simulink model "EGRVlv_VDPosGov"  (R2018a)
settings: configuration reference "cs_ert" (kept outside this file)
model workspace (MAT data in the model file):
  EGRVlv_VDPosGov_DT = 10
values from neighbouring files (symbols this model uses):
  EGRVlv_DKdNgv_C = -5.0    [EGRVlv_VDPosGov.sldd]
  EGRVlv_DKdPsv_C = 5.0    [EGRVlv_VDPosGov.sldd]
  EGRVlv_facCrntEffFlt_C = 50.0    [EGRVlv_VDPosGov.sldd]
  EGRVlv_iEff_CUR : value not decoded    [EGRVlv_VDPosGov.sldd]
  EGRVlv_iEff_CURX : value not decoded    [EGRVlv_VDPosGov.sldd]
  EGRVlv_iEffOvrLd_C = 200.0    [EGRVlv_VDPosGov.sldd]
  EGRVlv_rDesEGR_CUR : value not decoded    [EGRVlv_VDPosGov.sldd]
  EGRVlv_rDesEGR_CURX : value not decoded    [EGRVlv_VDPosGov.sldd]
  EGRVlv_rEGRDflVal_C = 0.0    [EGRVlv_VDPosGov.sldd]
  EGRVlv_rEGRSwtOff_C = 20.0    [EGRVlv_VDPosGov.sldd]
  EGRVlv_rGovDvtThres_C = 30.0    [EGRVlv_VDPosGov.sldd]
  EGRVlv_rGovMax_C = 30.0    [EGRVlv_VDPosGov.sldd]
  EGRVlv_rGovMax_CUR : value not decoded    [EGRVlv_VDPosGov.sldd]
  EGRVlv_rGovMax_CURX : value not decoded    [EGRVlv_VDPosGov.sldd]
  EGRVlv_rGovMin_C = 10.0    [EGRVlv_VDPosGov.sldd]
  EGRVlv_rGovMin_CUR : value not decoded    [EGRVlv_VDPosGov.sldd]
  EGRVlv_rGovMin_CURX : value not decoded    [EGRVlv_VDPosGov.sldd]
  EGRVlv_rIniStp_C = 5.0    [EGRVlv_VDPosGov.sldd]
  EGRVlv_rOutIMax_C = 30.0    [EGRVlv_VDPosGov.sldd]
  EGRVlv_rPIDWinNgv_C = -10.0    [EGRVlv_VDPosGov.sldd]
  EGRVlv_rPIDWinPsv_C = 10.0    [EGRVlv_VDPosGov.sldd]
  EGRVlv_rSwtOffRmp_C = 2.0    [EGRVlv_VDPosGov.sldd]
  EGRVlv_SlwClsDKd_C = 3.0    [EGRVlv_VDPosGov.sldd]
  EGRVlv_SlwClsIKi_C = 0.2    [EGRVlv_VDPosGov.sldd]
  EGRVlv_SlwClsPKp_C = 3.0    [EGRVlv_VDPosGov.sldd]
  EGRVlv_SmlSigNgvDKd_C = -5.0    [EGRVlv_VDPosGov.sldd]
  EGRVlv_SmlSigNgvIKi_C = -1.0    [EGRVlv_VDPosGov.sldd]
  EGRVlv_SmlSigNgvPKp_C = -5.0    [EGRVlv_VDPosGov.sldd]
  EGRVlv_SmlSigPsvDKd_C = 5.0    [EGRVlv_VDPosGov.sldd]
  EGRVlv_SmlSigPsvIKi_C = 1.0    [EGRVlv_VDPosGov.sldd]
  EGRVlv_SmlSigPsvPKp_C = 5.0    [EGRVlv_VDPosGov.sldd]
  EGRVlv_swtDesValNrmInv_C = 1.0    [EGRVlv_VDPosGov.sldd]
  EGRVlv_swtGovByp_C = 0.0    [EGRVlv_VDPosGov.sldd]
  EGRVlv_tiLimDlyOvrLd_C = 1.0    [EGRVlv_VDPosGov.sldd]
  EGRVlv_tiOutIMax_C = 1.0    [EGRVlv_VDPosGov.sldd]
undefined symbols (not defined in the file or in its folder): CEngDsT_tTransf_CURX
libraries: simulink x10, sllib x5
settings Model: DataDictionary=EGRVlv_VDPosGov.sldd  Creator=zhoutinglin  LastModifiedBy=zhoutinglin

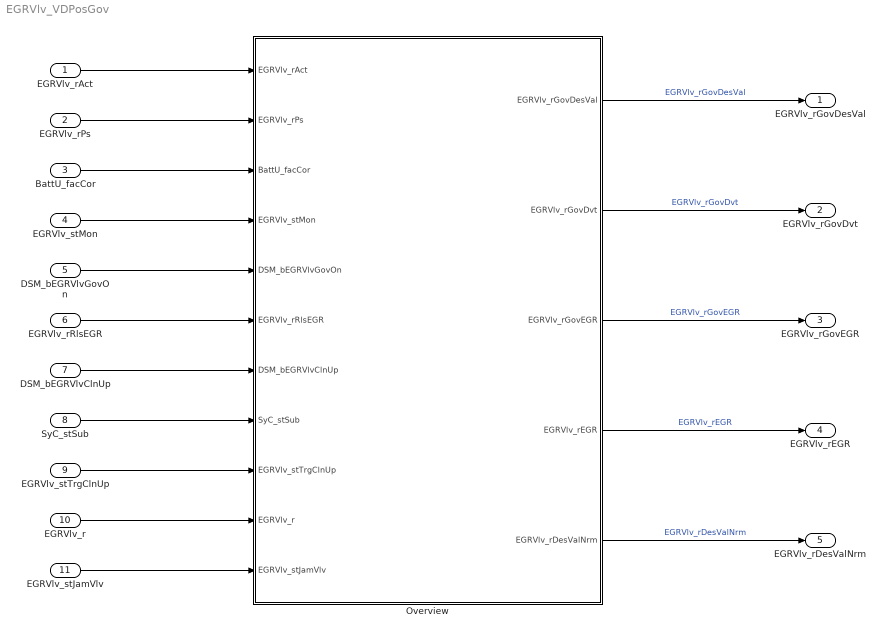
== system EGRVlv_VDPosGov ==
  EGRVlv_rAct : Inport  Description=Commanded value from application SW  OutMin=-100  OutMax=100  OutDataTypeStr=DutyCycle  Unit=%  PortDimensions=[1 1]
  EGRVlv_rPs : Inport  Description=Actuatorposition  Port=2  OutMin=-100  OutMax=100  OutDataTypeStr=DutyCycle  Unit=%  PortDimensions=[1 1]
  BattU_facCor : Inport  Description=Additional control value to release a jammed valve  Port=3  OutMin=-32  OutMax=31.9  OutDataTypeStr=Fac_100  PortDimensions=[1 1]
  EGRVlv_stMon : Inport  Description=Duty cycle to power stage  Port=4  OutMin=0  OutMax=65535  OutDataTypeStr=State2  PortDimensions=[1 1]
  DSM_bEGRVlvGovOn : Inport  Description=Battery correction factor  Port=5  OutMin=0  OutMax=1  OutDataTypeStr=boolean  PortDimensions=[1 1]
  EGRVlv_rRlsEGR : Inport  Description=State of system monitoring  Port=6  OutMin=-100  OutMax=100  OutDataTypeStr=DutyCycle  PortDimensions=[1 1]
  DSM_bEGRVlvClnUp : Inport  Description=Status of FId_EGRVlvGovOn  Port=7  OutMin=0  OutMax=1  OutDataTypeStr=boolean  PortDimensions=[1 1]
  SyC_stSub : Inport  Description=Status of offset learning  Port=8  OutDataTypeStr=Enum: ECUPowerState  PortDimensions=[1 1]
  EGRVlv_stTrgClnUp : Inport  Description=Valve position (offset corrected without error handling)  Port=9  OutMin=0  OutMax=1  OutDataTypeStr=boolean  PortDimensions=[1 1]
  EGRVlv_r : Inport  Description=Status of FId_EGRVlvClnUp  Port=10  OutMin=-100  OutMax=100  OutDataTypeStr=DutyCycle  PortDimensions=[1 1]
  EGRVlv_stJamVlv : Inport  Description=Current system/ECU sub-state  Port=11  OutMin=0  OutMax=1  OutDataTypeStr=boolean  PortDimensions=[1 1]
  Overview : Subsystem
  EGRVlv_rGovDesVal : Outport
  EGRVlv_rGovDvt : Outport  Port=2
  EGRVlv_rGovEGR : Outport  Port=3
  EGRVlv_rEGR : Outport  Port=4
  EGRVlv_rDesValNrm : Outport  Port=5
  wires:
  EGRVlv_rAct/1 -> Overview/1(EGRVlv_rAct)
  EGRVlv_rPs/1 -> Overview/2(EGRVlv_rPs)
  BattU_facCor/1 -> Overview/3(BattU_facCor)
  EGRVlv_stMon/1 -> Overview/4(EGRVlv_stMon)
  DSM_bEGRVlvGovOn/1 -> Overview/5(DSM_bEGRVlvGovOn)
  EGRVlv_rRlsEGR/1 -> Overview/6(EGRVlv_rRlsEGR)
  DSM_bEGRVlvClnUp/1 -> Overview/7(DSM_bEGRVlvClnUp)
  SyC_stSub/1 -> Overview/8(SyC_stSub)
  EGRVlv_stTrgClnUp/1 -> Overview/9(EGRVlv_stTrgClnUp)
  EGRVlv_r/1 -> Overview/10(EGRVlv_r)
  EGRVlv_stJamVlv/1 -> Overview/11(EGRVlv_stJamVlv)
  Overview/1(EGRVlv_rGovDesVal) -> EGRVlv_rGovDesVal/1  "EGRVlv_rGovDesVal"
  Overview/2(EGRVlv_rGovDvt) -> EGRVlv_rGovDvt/1  "EGRVlv_rGovDvt"
  Overview/3(EGRVlv_rGovEGR) -> EGRVlv_rGovEGR/1  "EGRVlv_rGovEGR"
  Overview/4(EGRVlv_rEGR) -> EGRVlv_rEGR/1  "EGRVlv_rEGR"
  Overview/5(EGRVlv_rDesValNrm) -> EGRVlv_rDesValNrm/1  "EGRVlv_rDesValNrm"

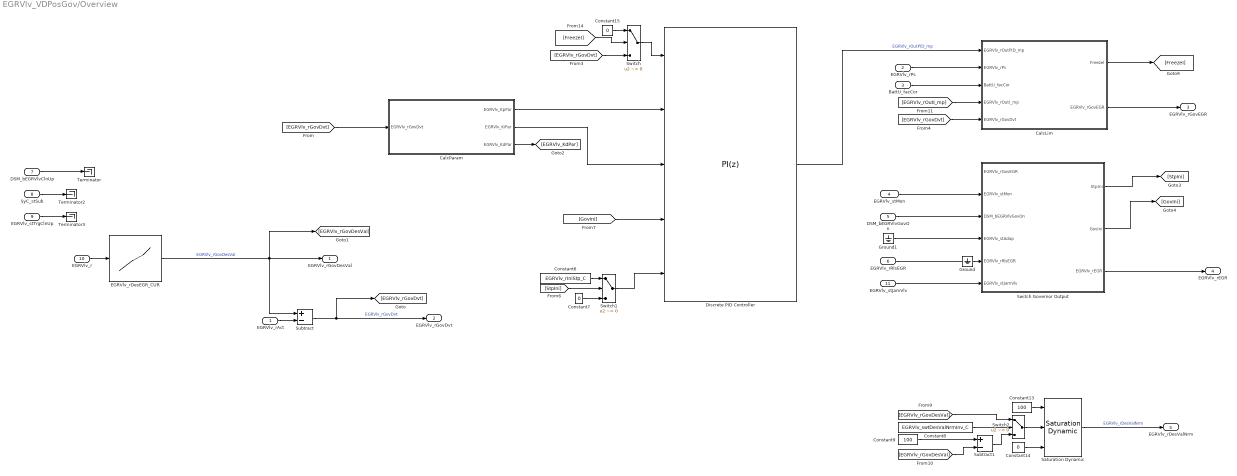
== system EGRVlv_VDPosGov/Overview ==
  EGRVlv_rAct : Inport  Tag=%
  EGRVlv_rPs : Inport  Tag=%  Port=2
  BattU_facCor : Inport  Tag=%  Port=3
  EGRVlv_stMon : Inport  Tag=%  Port=4
  DSM_bEGRVlvGovOn : Inport  Tag=%  Port=5
  EGRVlv_rRlsEGR : Inport  Tag=%  Port=6
  DSM_bEGRVlvClnUp : Inport  Tag=%  Port=7
  SyC_stSub : Inport  Tag=%  Port=8
  EGRVlv_stTrgClnUp : Inport  Tag=%  Port=9
  EGRVlv_r : Inport  Tag=%  Port=10
  EGRVlv_stJamVlv : Inport  Port=11
  CalcLim : Subsystem
  CalcParam : Subsystem
  Constant13 : Constant  Value=100  OutDataTypeStr=Inherit: Inherit via back propagation
  Constant14 : Constant  Value=0  OutDataTypeStr=Inherit: Inherit via back propagation
  Constant15 : Constant  Value=0  OutDataTypeStr=Inherit: Inherit via back propagation
  Constant6 : Constant  Value=EGRVlv_rIniStp_C
  Constant7 : Constant  Value=0  OutDataTypeStr=Inherit: Inherit via back propagation
  Constant8 : Constant  Value=EGRVlv_swtDesValNrmInv_C
  Constant9 : Constant  Value=100  OutDataTypeStr=Inherit: Inherit via back propagation
  Discrete PID Controller : simulink/Continuous/PID Controller  Controller=PI  TimeDomain=Discrete-time  SampleTime=-1  IntegratorMethod=Forward Euler  FilterMethod=Forward Euler  Form=Parallel  UseFilter=on  ControllerParametersSource=external  P=1  I=1  D=0  N=100  InitialConditionSource=external  InitialConditionForIntegrator=0  InitialConditionForFilter=0  ExternalReset=level  ZeroCross=off  LimitOutput=off  UpperSaturationLimit=inf  LowerSaturationLimit=-inf  LinearizeAsGain=off  AntiWindupMode=none  Kb=1  TrackingMode=off  Kt=1  SaturateOnIntegerOverflow=on  PParamMin=[]  PParamMax=[]  IParamMin=[]  IParamMax=[]  DParamMin=[]  DParamMax=[]  NParamMin=[]  NParamMax=[]  KbParamMin=[]  KbParamMax=[]  KtParamMin=[]  KtParamMax=[]  POutMin=[]  POutMax=[]  IOutMin=[]  IOutMax=[]  DOutMin=[]  DOutMax=[]  NOutMin=[]  NOutMax=[]  KbOutMin=[]  KbOutMax=[]  KtOutMin=[]  KtOutMax=[]  IntegratorOutMin=[]  IntegratorOutMax=[]  FilterOutMin=[]  FilterOutMax=[]  SumOutMin=[]  SumOutMax=[]  SumOutDataTypeStr=Inherit: Inherit via back propagation  SumI1OutMin=[]  SumI1OutMax=[]  SumI2OutMin=[]  SumI2OutMax=[]  SumI3OutMin=[]  SumI3OutMax=[]  SumDOutMin=[]  SumDOutMax=[]  SaturationOutMin=[]  SaturationOutMax=[]  IntegratorContinuousStateAttributes=''  IntegratorStateMustResolveToSignalObject=off  IntegratorRTWStateStorageClass=Auto  FilterContinuousStateAttributes=''  FilterStateMustResolveToSignalObject=off  FilterRTWStateStorageClass=Auto  DifferentiatorICPrevScaledInput=0  DifferentiatorOutMin=[]  DifferentiatorOutMax=[]  FilterDiffOutCoefMin=[]  FilterDiffOutCoefMax=[]  SumDenOutMin=[]  SumDenOutMax=[]  SumNumOutMin=[]  SumNumOutMax=[]  ReciprocalOutMin=[]  ReciprocalOutMax=[]  DivideOutMin=[]  DivideOutMax=[]  TunerSelectOption=Transfer Function Based (PID Tuner App)
  EGRVlv_rDesEGR_CUR : Lookup_n-D  DialogController=Simulink.DDGSource  NumberOfTableDimensions=1  BreakpointsForDimension1=EGRVlv_rDesEGR_CURX  BreakpointsForDimension2=CEngDsT_tTransf_CURX  IndexSearchMethod=Linear search  BeginIndexSearchUsingPreviousIndexResult=on  Table=EGRVlv_rDesEGR_CUR  TableDataTypeStr=Inherit: Inherit from 'Table data'  ExtrapMethod=Clip  UseLastTableValue=on  InternalRulePriority=Speed  OutDataTypeStr=Inherit: Inherit from 'Table data'  SaturateOnIntegerOverflow=on
  Ground : Ground
  Ground1 : Ground
  Saturation Dynamic : simulink/Discontinuities/Saturation Dynamic  OutMin=[]  OutMax=[]  OutDataTypeStr=Inherit: Same as second input  OutDataType=fixdt(1, 16)  OutScaling=2^-10  DoSatur=off
  Subtract : Sum  Inputs=+-  SaturateOnIntegerOverflow=on
  Subtract1 : Sum  Inputs=+-  SaturateOnIntegerOverflow=on  InputSameDT=on
  Switch : Switch  Criteria=u2 ~= 0
  Switch Governor Output : Subsystem
  Switch1 : Switch  Criteria=u2 ~= 0
  Switch2 : Switch  Criteria=u2 ~= 0  InputSameDT=on
  Terminator : Terminator
  Terminator2 : Terminator
  Terminator3 : Terminator
  EGRVlv_rGovDesVal : Outport  Tag=%
  EGRVlv_rGovDvt : Outport  Tag=%  Port=2
  EGRVlv_rGovEGR : Outport  Tag=%  Port=3
  EGRVlv_rEGR : Outport  Tag=%  Port=4
  EGRVlv_rDesValNrm : Outport  Tag=%  Port=5
  wires:
  [EGRVlv_rGovDvt] -> CalcLim/5(EGRVlv_rGovDvt)
  CalcParam/1(EGRVlv_KpPar) -> Discrete PID Controller/2
  Saturation Dynamic/1 -> EGRVlv_rDesValNrm/1  "EGRVlv_rDesValNrm"
  CalcLim/1(Freezel) -> [FreezeI]
  Switch1/1 -> Discrete PID Controller/5
  Switch/1 -> Discrete PID Controller/1
  Constant14/1 -> Saturation Dynamic/3
  [GovIni] -> Discrete PID Controller/4
  Subtract1/1 -> Switch2/3
  Switch2/1 -> Saturation Dynamic/2
  [FreezeI] -> Switch/2
  Switch Governor Output/2(GovIni) -> [GovIni]
  [EGRVlv_rGovDvt] -> CalcParam/1(EGRVlv_rGovDvt)
  [EGRVlv_rOutI_mp] -> CalcLim/4(EGRVlv_rOutI_mp)
  Switch Governor Output/1(StpIni) -> [StpIni]
  DSM_bEGRVlvClnUp/1 -> Terminator/1
  Constant9/1 -> Subtract1/1
  SyC_stSub/1 -> Terminator2/1
  EGRVlv_stTrgClnUp/1 -> Terminator3/1
  Constant15/1 -> Switch/1
  [StpIni] -> Switch1/2
  Constant6/1 -> Switch1/1
  Constant7/1 -> Switch1/3
  Constant13/1 -> Saturation Dynamic/1
  Discrete PID Controller/1 -> CalcLim/1(EGRVlv_rOutPID_mp)  "EGRVlv_rOutPID_mp"
  CalcParam/3(EGRVlv_KdPar) -> [EGRVlv_KdPar]
  EGRVlv_rDesEGR_CUR/1 -> [EGRVlv_rGovDesVal], EGRVlv_rGovDesVal/1, Subtract/1  "EGRVlv_rGovDesVal"
  [EGRVlv_rGovDesVal] -> Subtract1/2
  CalcParam/2(EGRVlv_KiPar) -> Discrete PID Controller/3
  [EGRVlv_rGovDesVal] -> Switch2/1
  [EGRVlv_rGovDvt] -> Switch/3
  BattU_facCor/1 -> CalcLim/3(BattU_facCor)
  CalcLim/2(EGRVlv_rGovEGR) -> EGRVlv_rGovEGR/1
  EGRVlv_rPs/1 -> CalcLim/2(EGRVlv_rPs)
  EGRVlv_rAct/1 -> Subtract/2
  Subtract/1 -> EGRVlv_rGovDvt/1, [EGRVlv_rGovDvt]  "EGRVlv_rGovDvt"
  Constant8/1 -> Switch2/2
  EGRVlv_r/1 -> EGRVlv_rDesEGR_CUR/1
  Ground/1 -> ?
  EGRVlv_stMon/1 -> Switch Governor Output/2(EGRVlv_stMon)
  DSM_bEGRVlvGovOn/1 -> Switch Governor Output/3(DSM_bEGRVlvGovOn)
  Ground1/1 -> Switch Governor Output/4(EGRVlv_stAdap)
  EGRVlv_rRlsEGR/1 -> Switch Governor Output/5(EGRVlv_rRlsEGR)
  EGRVlv_stJamVlv/1 -> Switch Governor Output/6(EGRVlv_stJamVlv)
  Switch Governor Output/3(EGRVlv_rEGR) -> EGRVlv_rEGR/1

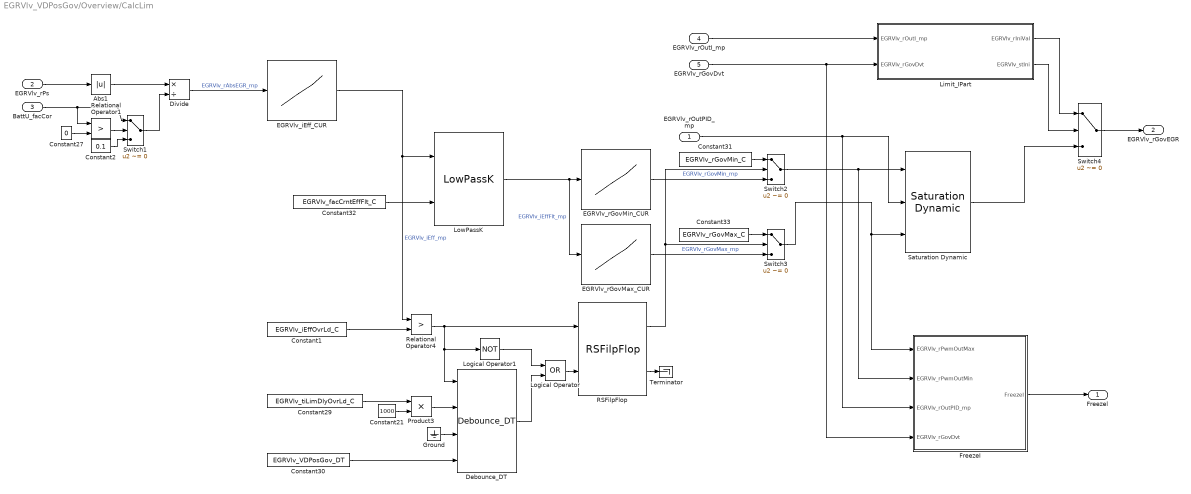
== system EGRVlv_VDPosGov/Overview/CalcLim ==
  EGRVlv_rOutPID_mp : Inport  Tag=%
  EGRVlv_rPs : Inport  Tag=%  Port=2
  BattU_facCor : Inport  Tag=%  Port=3
  EGRVlv_rOutI_mp : Inport  Tag=%  Port=4
  EGRVlv_rGovDvt : Inport  Tag=%  Port=5
  Abs1 : Abs
  Constant1 : Constant  Value=EGRVlv_iEffOvrLd_C
  Constant2 : Constant  Value=0.1  OutDataTypeStr=Inherit: Inherit via back propagation
  Constant21 : Constant  Value=1000  OutDataTypeStr=uint16
  Constant27 : Constant  Value=0  OutDataTypeStr=Inherit: Inherit via back propagation
  Constant29 : Constant  Value=EGRVlv_tiLimDlyOvrLd_C
  Constant30 : Constant  Value=EGRVlv_VDPosGov_DT  OutDataTypeStr=Inherit: Inherit via back propagation
  Constant31 : Constant  Value=EGRVlv_rGovMin_C
  Constant32 : Constant  Value=EGRVlv_facCrntEffFlt_C
  Constant33 : Constant  Value=EGRVlv_rGovMax_C
  Debounce_DT : sllib/Debounce_DT
      settings: SourceProductName=sllib
  Divide : Product  Inputs=*/  OutDataTypeStr=Inherit: Inherit via back propagation  SaturateOnIntegerOverflow=on
  EGRVlv_iEff_CUR : Lookup_n-D  DialogController=Simulink.DDGSource  NumberOfTableDimensions=1  BreakpointsForDimension1=EGRVlv_iEff_CURX  BreakpointsForDimension2=CEngDsT_tTransf_CURX  IndexSearchMethod=Linear search  BeginIndexSearchUsingPreviousIndexResult=on  Table=EGRVlv_iEff_CUR  TableDataTypeStr=Inherit: Inherit from 'Table data'  ExtrapMethod=Clip  UseLastTableValue=on  InternalRulePriority=Speed  OutDataTypeStr=Inherit: Inherit from 'Table data'  SaturateOnIntegerOverflow=on
  EGRVlv_rGovMax_CUR : Lookup_n-D  DialogController=Simulink.DDGSource  NumberOfTableDimensions=1  BreakpointsForDimension1=EGRVlv_rGovMax_CURX  BreakpointsForDimension2=CEngDsT_tTransf_CURX  IndexSearchMethod=Linear search  BeginIndexSearchUsingPreviousIndexResult=on  Table=EGRVlv_rGovMax_CUR  TableDataTypeStr=Inherit: Inherit from 'Table data'  ExtrapMethod=Clip  UseLastTableValue=on  InternalRulePriority=Speed  OutDataTypeStr=Inherit: Inherit from 'Table data'  SaturateOnIntegerOverflow=on
  EGRVlv_rGovMin_CUR : Lookup_n-D  DialogController=Simulink.DDGSource  NumberOfTableDimensions=1  BreakpointsForDimension1=EGRVlv_rGovMin_CURX  BreakpointsForDimension2=CEngDsT_tTransf_CURX  IndexSearchMethod=Linear search  BeginIndexSearchUsingPreviousIndexResult=on  Table=EGRVlv_rGovMin_CUR  TableDataTypeStr=Inherit: Inherit from 'Table data'  ExtrapMethod=Clip  UseLastTableValue=on  InternalRulePriority=Speed  OutDataTypeStr=Inherit: Inherit from 'Table data'  SaturateOnIntegerOverflow=on
  FreezeI : Subsystem
  Ground : Ground
  Limit_IPart : Subsystem
  Logical Operator : Logic  Operator=OR  AllPortsSameDT=off  OutDataTypeStr=boolean
  Logical Operator1 : Logic  Operator=NOT  AllPortsSameDT=off  OutDataTypeStr=boolean
  LowPassK : sllib/LowPassK
      settings: SourceProductName=sllib
  Product3 : Product  OutDataTypeStr=uint32  SaturateOnIntegerOverflow=on
  RSFilpFlop : sllib/RSFilpFlop
      settings: SourceProductName=sllib
  Relational Operator1 : RelationalOperator  Operator=>  OutDataTypeStr=boolean  RndMeth=Simplest  InputSameDT=on
  Relational Operator4 : RelationalOperator  Operator=>  OutDataTypeStr=boolean  RndMeth=Simplest
  Saturation Dynamic : simulink/Discontinuities/Saturation Dynamic  OutMin=[]  OutMax=[]  OutDataTypeStr=Inherit: Same as second input  OutDataType=fixdt(1, 16)  OutScaling=2^-10  DoSatur=off
  Switch{1..4} (4 alike) : Switch  Criteria=u2 ~= 0
  Terminator : Terminator
  Freezel : Outport
  EGRVlv_rGovEGR : Outport  Tag=%  Port=2
  wires:
  Abs1/1 -> Divide/1
  Constant33/1 -> Switch3/1
  RSFilpFlop/1 -> Switch3/2, Switch2/2
  EGRVlv_rGovMax_CUR/1 -> Switch3/3  "EGRVlv_rGovMax_mp"
  Switch2/1 -> Saturation Dynamic/1, FreezeI/2(EGRVlv_rPwmOutMin)
  Switch3/1 -> Saturation Dynamic/3, FreezeI/1(EGRVlv_rPwmOutMax)
  Debounce_DT/1 -> Logical Operator/2
  Logical Operator/1 -> RSFilpFlop/2
  Logical Operator1/1 -> Logical Operator/1
  Constant31/1 -> Switch2/1
  EGRVlv_iEff_CUR/1 -> Relational Operator4/1, LowPassK/1  "EGRVlv_iEff_mp"
  EGRVlv_rGovMin_CUR/1 -> Switch2/3  "EGRVlv_rGovMin_mp"
  Constant1/1 -> Relational Operator4/2
  Relational Operator4/1 -> RSFilpFlop/1, Debounce_DT/1, Logical Operator1/1
  EGRVlv_rPs/1 -> Abs1/1
  Divide/1 -> EGRVlv_iEff_CUR/1  "EGRVlv_rAbsEGR_mp"
  LowPassK/1 -> EGRVlv_rGovMax_CUR/1, EGRVlv_rGovMin_CUR/1  "EGRVlv_iEffFlt_mp"
  Constant29/1 -> Product3/1
  Constant30/1 -> Debounce_DT/4
  BattU_facCor/1 -> Relational Operator1/1, Switch1/1
  Constant32/1 -> LowPassK/2
  Relational Operator1/1 -> Switch1/2
  Constant27/1 -> Relational Operator1/2
  Constant2/1 -> Switch1/3
  Switch1/1 -> Divide/2
  Product3/1 -> Debounce_DT/2
  Limit_IPart/1(EGRVlv_rIniVal) -> Switch4/1
  Limit_IPart/2(EGRVlv_stIni) -> Switch4/2
  Switch4/1 -> EGRVlv_rGovEGR/1
  Saturation Dynamic/1 -> Switch4/3
  Constant21/1 -> Product3/2
  EGRVlv_rOutPID_mp/1 -> Saturation Dynamic/2, FreezeI/3(EGRVlv_rOutPID_mp)
  RSFilpFlop/2 -> Terminator/1
  EGRVlv_rOutI_mp/1 -> Limit_IPart/1(EGRVlv_rOutI_mp)
  EGRVlv_rGovDvt/1 -> Limit_IPart/2(EGRVlv_rGovDvt), FreezeI/4(EGRVlv_rGovDvt)
  FreezeI/1(FreezeI) -> Freezel/1
  Ground/1 -> Debounce_DT/3

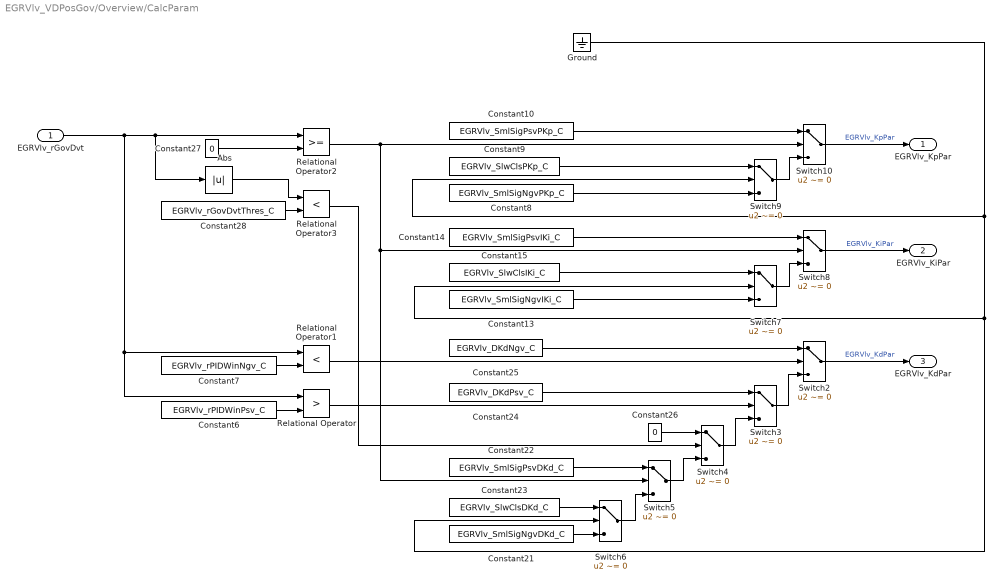
== system EGRVlv_VDPosGov/Overview/CalcParam ==
  EGRVlv_rGovDvt : Inport  Tag=%
  Abs : Abs
  Constant10 : Constant  Value=EGRVlv_SmlSigPsvPKp_C
  Constant13 : Constant  Value=EGRVlv_SmlSigNgvIKi_C
  Constant14 : Constant  Value=EGRVlv_SmlSigPsvIKi_C
  Constant15 : Constant  Value=EGRVlv_SlwClsIKi_C
  Constant21 : Constant  Value=EGRVlv_SmlSigNgvDKd_C
  Constant22 : Constant  Value=EGRVlv_SmlSigPsvDKd_C
  Constant23 : Constant  Value=EGRVlv_SlwClsDKd_C
  Constant24 : Constant  Value=EGRVlv_DKdPsv_C
  Constant25 : Constant  Value=EGRVlv_DKdNgv_C
  Constant26 : Constant  Value=0  OutDataTypeStr=Inherit: Inherit via back propagation
  Constant27 : Constant  Value=0  OutDataTypeStr=Inherit: Inherit via back propagation
  Constant28 : Constant  Value=EGRVlv_rGovDvtThres_C
  Constant6 : Constant  Value=EGRVlv_rPIDWinPsv_C
  Constant7 : Constant  Value=EGRVlv_rPIDWinNgv_C
  Constant8 : Constant  Value=EGRVlv_SmlSigNgvPKp_C
  Constant9 : Constant  Value=EGRVlv_SlwClsPKp_C
  Ground : Ground
  Relational Operator : RelationalOperator  Operator=>  OutDataTypeStr=boolean  RndMeth=Simplest
  Relational Operator1 : RelationalOperator  Operator=<  OutDataTypeStr=boolean  RndMeth=Simplest
  Relational Operator2 : RelationalOperator  OutDataTypeStr=boolean  RndMeth=Simplest  InputSameDT=on
  Relational Operator3 : RelationalOperator  Operator=<  OutDataTypeStr=boolean  RndMeth=Simplest
  Switch{2..10} (9 alike) : Switch  Criteria=u2 ~= 0
  EGRVlv_KpPar : Outport  Tag=%
  EGRVlv_KiPar : Outport  Tag=%  Port=2
  EGRVlv_KdPar : Outport  Tag=%  Port=3
  wires:
  Constant6/1 -> Relational Operator/2
  EGRVlv_rGovDvt/1 -> Relational Operator2/1, Abs/1, Relational Operator1/1, Relational Operator/1
  Constant7/1 -> Relational Operator1/2
  Abs/1 -> Relational Operator3/1
  Constant27/1 -> Relational Operator2/2
  Constant28/1 -> Relational Operator3/2
  Relational Operator1/1 -> Switch2/2
  Constant25/1 -> Switch2/1
  Switch3/1 -> Switch2/3
  Relational Operator/1 -> Switch3/2
  Constant24/1 -> Switch3/1
  Switch4/1 -> Switch3/3
  Relational Operator3/1 -> Switch4/2
  Constant26/1 -> Switch4/1
  Switch5/1 -> Switch4/3
  Relational Operator2/1 -> Switch10/2, Switch8/2, Switch5/2
  Constant22/1 -> Switch5/1
  Switch6/1 -> Switch5/3
  Constant23/1 -> Switch6/1
  Constant21/1 -> Switch6/3
  Switch7/1 -> Switch8/3
  Constant14/1 -> Switch8/1
  Constant15/1 -> Switch7/1
  Constant13/1 -> Switch7/3
  Ground/1 -> Switch6/2, Switch7/2, Switch9/2
  Switch9/1 -> Switch10/3
  Constant10/1 -> Switch10/1
  Constant9/1 -> Switch9/1
  Constant8/1 -> Switch9/3
  Switch10/1 -> EGRVlv_KpPar/1  "EGRVlv_KpPar"
  Switch8/1 -> EGRVlv_KiPar/1  "EGRVlv_KiPar"
  Switch2/1 -> EGRVlv_KdPar/1  "EGRVlv_KdPar"

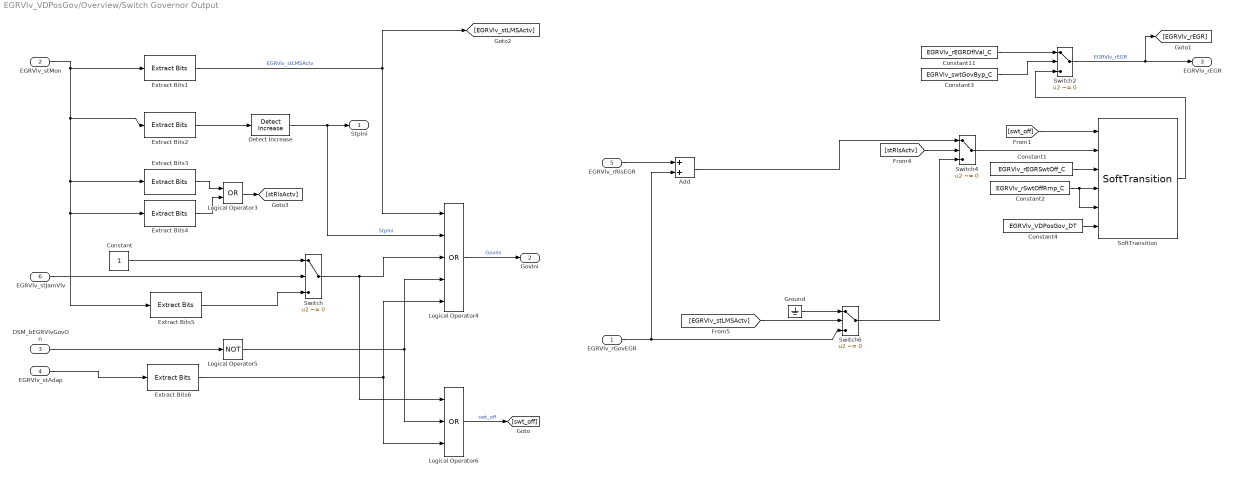
== system EGRVlv_VDPosGov/Overview/Switch Governor Output ==
  EGRVlv_rGovEGR : Inport  Tag=%
  EGRVlv_stMon : Inport  Tag=%  Port=2
  DSM_bEGRVlvGovOn : Inport  Tag=%  Port=3
  EGRVlv_stAdap : Inport  Tag=%  Port=4
  EGRVlv_rRlsEGR : Inport  Tag=%  Port=5
  EGRVlv_stJamVlv : Inport  Port=6
  Add : Sum  SaturateOnIntegerOverflow=on
  Constant : Constant  OutDataTypeStr=boolean
  Constant1 : Constant  Value=EGRVlv_rEGRSwtOff_C
  Constant11 : Constant  Value=EGRVlv_rEGRDflVal_C
  Constant2 : Constant  Value=EGRVlv_rSwtOffRmp_C
  Constant3 : Constant  Value=EGRVlv_swtGovByp_C
  Constant4 : Constant  Value=EGRVlv_VDPosGov_DT  OutDataTypeStr=Inherit: Inherit via back propagation
  Detect Increase : simulink/Logic and Bit Operations/Detect Increase  vinit=0.0  OutDataTypeStr=boolean
  Extract Bits1 : simulink/Logic and Bit Operations/Extract Bits  bitsToExtract=Range of bits  numBits=8  bitIdxRange=[0 0]  outScalingMode=Treat bit field as an integer
      settings: SourceProductName=Simulink
  Extract Bits2 : simulink/Logic and Bit Operations/Extract Bits  bitsToExtract=Range of bits  numBits=8  bitIdxRange=[4 4]  outScalingMode=Treat bit field as an integer
      settings: SourceProductName=Simulink
  Extract Bits3 : simulink/Logic and Bit Operations/Extract Bits  bitsToExtract=Range of bits  numBits=8  bitIdxRange=[6 6]  outScalingMode=Treat bit field as an integer
      settings: SourceProductName=Simulink
  Extract Bits4 : simulink/Logic and Bit Operations/Extract Bits  bitsToExtract=Range of bits  numBits=8  bitIdxRange=[8 8]  outScalingMode=Treat bit field as an integer
      settings: SourceProductName=Simulink
  Extract Bits5 : simulink/Logic and Bit Operations/Extract Bits  bitsToExtract=Range of bits  numBits=8  bitIdxRange=[10 10]  outScalingMode=Treat bit field as an integer
      settings: SourceProductName=Simulink
  Extract Bits6 : simulink/Logic and Bit Operations/Extract Bits  bitsToExtract=Range of bits  numBits=8  bitIdxRange=[0 0]  outScalingMode=Treat bit field as an integer
      settings: SourceProductName=Simulink
  Ground : Ground
  Logical Operator3 : Logic  Operator=OR  AllPortsSameDT=off  OutDataTypeStr=boolean
  Logical Operator4 : Logic  Operator=OR  Inputs=5  AllPortsSameDT=off  OutDataTypeStr=boolean
  Logical Operator5 : Logic  Operator=NOT  AllPortsSameDT=off  OutDataTypeStr=boolean
  Logical Operator6 : Logic  Operator=OR  Inputs=3  AllPortsSameDT=off  OutDataTypeStr=boolean
  SoftTransition : sllib/SoftTransition
      settings: SourceProductName=sllib
  Switch{,2,4,6} (4 alike) : Switch  Criteria=u2 ~= 0
  StpIni : Outport  Tag=%
  GovIni : Outport  Tag=%  Port=2
  EGRVlv_rEGR : Outport  Tag=%  Port=3
  wires:
  Logical Operator4/1 -> GovIni/1  "GovIni"
  Logical Operator5/1 -> Logical Operator4/4, Logical Operator6/2
  DSM_bEGRVlvGovOn/1 -> Logical Operator5/1
  Detect Increase/1 -> Logical Operator4/2, StpIni/1  "StpIni"
  Logical Operator6/1 -> [swt_off]  "swt_off"
  Extract Bits1/1 -> [EGRVlv_stLMSActv], Logical Operator4/1  "EGRVlv_stLMSActv"
  EGRVlv_rRlsEGR/1 -> Add/1
  EGRVlv_rGovEGR/1 -> Add/2, Switch6/3
  Switch2/1 -> EGRVlv_rEGR/1, [EGRVlv_rEGR]  "EGRVlv_rEGR"
  Constant2/1 -> SoftTransition/5, SoftTransition/4
  Ground/1 -> Switch6/1
  SoftTransition/1 -> Switch2/3
  Switch4/1 -> SoftTransition/2
  Switch6/1 -> Switch4/3
  Constant11/1 -> Switch2/1
  Constant3/1 -> Switch2/2
  [swt_off] -> SoftTransition/1
  Logical Operator3/1 -> [stRlsActv]
  [EGRVlv_stLMSActv] -> Switch6/2
  Extract Bits2/1 -> Detect Increase/1
  Extract Bits3/1 -> Logical Operator3/1
  Extract Bits4/1 -> Logical Operator3/2
  Extract Bits6/1 -> Logical Operator4/5, Logical Operator6/3
  EGRVlv_stMon/1 -> Extract Bits1/1, Extract Bits2/1, Extract Bits5/1, Extract Bits4/1, Extract Bits3/1
  Constant1/1 -> SoftTransition/3
  EGRVlv_stAdap/1 -> Extract Bits6/1
  [stRlsActv] -> Switch4/2
  Add/1 -> Switch4/1
  Constant/1 -> Switch/1
  EGRVlv_stJamVlv/1 -> Switch/2
  Extract Bits5/1 -> Switch/3
  Switch/1 -> Logical Operator6/1, Logical Operator4/3
  Constant4/1 -> SoftTransition/6

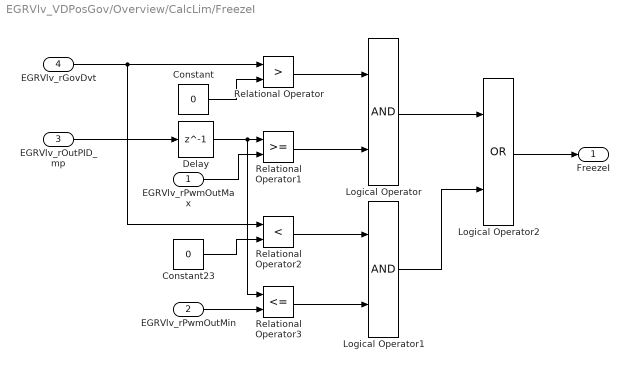
== system EGRVlv_VDPosGov/Overview/CalcLim/FreezeI ==
  EGRVlv_rPwmOutMax : Inport
  EGRVlv_rPwmOutMin : Inport  Port=2
  EGRVlv_rOutPID_mp : Inport  Port=3
  EGRVlv_rGovDvt : Inport  Port=4
  Constant : Constant  Value=0  OutDataTypeStr=Inherit: Inherit via back propagation
  Constant23 : Constant  Value=0  OutDataTypeStr=Inherit: Inherit via back propagation
  Delay : Delay  DelayLength=1  InitialCondition=0
  Logical Operator : Logic  AllPortsSameDT=off  OutDataTypeStr=boolean
  Logical Operator1 : Logic  AllPortsSameDT=off  OutDataTypeStr=boolean
  Logical Operator2 : Logic  Operator=OR  AllPortsSameDT=off  OutDataTypeStr=boolean
  Relational Operator : RelationalOperator  Operator=>  OutDataTypeStr=boolean  RndMeth=Simplest  InputSameDT=on
  Relational Operator1 : RelationalOperator  OutDataTypeStr=boolean  RndMeth=Simplest
  Relational Operator2 : RelationalOperator  Operator=<  OutDataTypeStr=boolean  RndMeth=Simplest  InputSameDT=on
  Relational Operator3 : RelationalOperator  Operator=<=  OutDataTypeStr=boolean  RndMeth=Simplest
  FreezeI : Outport
  wires:
  Logical Operator/1 -> Logical Operator2/1
  Logical Operator1/1 -> Logical Operator2/2
  Logical Operator2/1 -> FreezeI/1
  Relational Operator1/1 -> Logical Operator/2
  EGRVlv_rPwmOutMin/1 -> Relational Operator3/2
  Relational Operator2/1 -> Logical Operator1/1
  Relational Operator3/1 -> Logical Operator1/2
  EGRVlv_rPwmOutMax/1 -> Relational Operator1/2
  Constant/1 -> Relational Operator/2
  Constant23/1 -> Relational Operator2/2
  Delay/1 -> Relational Operator3/1, Relational Operator1/1
  EGRVlv_rGovDvt/1 -> Relational Operator/1, Relational Operator2/1
  Relational Operator/1 -> Logical Operator/1
  EGRVlv_rOutPID_mp/1 -> Delay/1

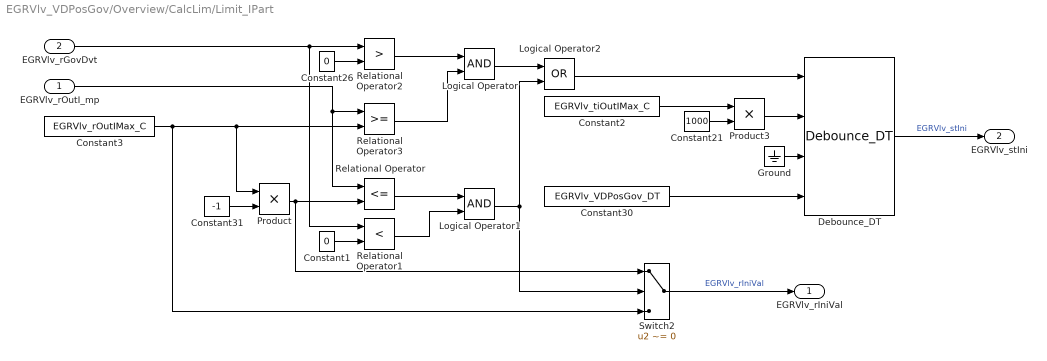
== system EGRVlv_VDPosGov/Overview/CalcLim/Limit_IPart ==
  EGRVlv_rOutI_mp : Inport  Tag=%
  EGRVlv_rGovDvt : Inport  Tag=%  Port=2
  Constant1 : Constant  Value=0  OutDataTypeStr=Inherit: Inherit via back propagation
  Constant2 : Constant  Value=EGRVlv_tiOutIMax_C
  Constant21 : Constant  Value=1000  OutDataTypeStr=uint16
  Constant26 : Constant  Value=0  OutDataTypeStr=Inherit: Inherit via back propagation
  Constant3 : Constant  Value=EGRVlv_rOutIMax_C
  Constant30 : Constant  Value=EGRVlv_VDPosGov_DT  OutDataTypeStr=Inherit: Inherit via back propagation
  Constant31 : Constant  Value=-1  OutDataTypeStr=int8
  Debounce_DT : sllib/Debounce_DT
      settings: SourceProductName=sllib
  Ground : Ground
  Logical Operator : Logic  AllPortsSameDT=off  OutDataTypeStr=boolean
  Logical Operator1 : Logic  AllPortsSameDT=off  OutDataTypeStr=boolean
  Logical Operator2 : Logic  Operator=OR  AllPortsSameDT=off  OutDataTypeStr=boolean
  Product : Product  OutDataTypeStr=Inherit: Inherit via back propagation  SaturateOnIntegerOverflow=on
  Product3 : Product  OutDataTypeStr=uint32  SaturateOnIntegerOverflow=on
  Relational Operator : RelationalOperator  Operator=<=  OutDataTypeStr=boolean  RndMeth=Simplest  InputSameDT=on
  Relational Operator1 : RelationalOperator  Operator=<  OutDataTypeStr=boolean  RndMeth=Simplest  InputSameDT=on
  Relational Operator2 : RelationalOperator  Operator=>  OutDataTypeStr=boolean  RndMeth=Simplest  InputSameDT=on
  Relational Operator3 : RelationalOperator  OutDataTypeStr=boolean  RndMeth=Simplest
  Switch2 : Switch  Criteria=u2 ~= 0
  EGRVlv_rIniVal : Outport  Tag=%
  EGRVlv_stIni : Outport  Tag=%  Port=2
  wires:
  Constant31/1 -> Product/2
  Constant30/1 -> Debounce_DT/4
  Relational Operator1/1 -> Logical Operator1/2
  EGRVlv_rGovDvt/1 -> Relational Operator2/1, Relational Operator1/1
  Constant26/1 -> Relational Operator2/2
  Relational Operator/1 -> Logical Operator1/1
  Constant1/1 -> Relational Operator1/2
  Logical Operator/1 -> Logical Operator2/1
  Relational Operator3/1 -> Logical Operator/2
  Constant2/1 -> Product3/1
  Relational Operator2/1 -> Logical Operator/1
  Logical Operator2/1 -> Debounce_DT/1
  EGRVlv_rOutI_mp/1 -> Relational Operator3/1, Relational Operator/1
  Product3/1 -> Debounce_DT/2
  Constant21/1 -> Product3/2
  Debounce_DT/1 -> EGRVlv_stIni/1  "EGRVlv_stIni"
  Product/1 -> Switch2/1, Relational Operator/2
  Logical Operator1/1 -> Logical Operator2/2, Switch2/2
  Constant3/1 -> Switch2/3, Product/1, Relational Operator3/2
  Switch2/1 -> EGRVlv_rIniVal/1  "EGRVlv_rIniVal"
  Ground/1 -> Debounce_DT/3
